simulink model "PPINFF"  (R2019a)
settings: Solver=VariableStepAuto  StartTime=0.0  StopTime=10.0  RelTol=1e-3
libraries: simulink x2
settings Model: Creator=pareshsoni  LastModifiedBy=pareshsoni

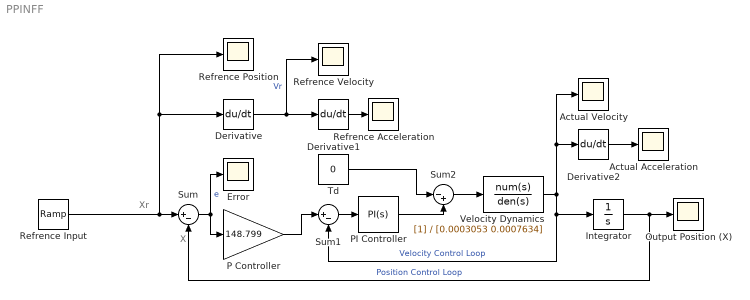
== system PPINFF ==
  note: X
  note: Xr
  Actual Acceleration : Scope
  Actual Velocity : Scope
  Derivative : Derivative  CoefficientInTFapproximation=0
  Derivative1 : Derivative
  Derivative2 : Derivative
  Error : Scope
  Integrator : Integrator
  Output Position (X) : Scope
  P Controller : Gain  Gain=148.799
  PI Controller : simulink/Continuous/PID Controller  Controller=PI  Form=Ideal  TimeDomain=Continuous-time  SampleTime=-1  IntegratorMethod=Forward Euler  FilterMethod=Forward Euler  ControllerParametersSource=internal  P=0.1296  I=25.1332  D=0  UseFilter=on  N=100  TunerSelectOption=Transfer Function Based (PID Tuner App)  InitialConditionSource=internal  InitialConditionForIntegrator=0  InitialConditionForFilter=0  DifferentiatorICPrevScaledInput=0  ExternalReset=none  TrackingMode=off  Kt=1  LimitOutput=off  UpperSaturationLimit=inf  LowerSaturationLimit=-inf  LinearizeAsGain=on  AntiWindupMode=none  Kb=1  POutMin=[]  POutMax=[]  IOutMin=[]  IOutMax=[]  DOutMin=[]  DOutMax=[]  NOutMin=[]  NOutMax=[]  SumOutMin=[]  SumOutMax=[]  SaturationOutMin=[]  SaturationOutMax=[]  PParamMin=[]  PParamMax=[]  IParamMin=[]  IParamMax=[]  DParamMin=[]  DParamMax=[]  NParamMin=[]  NParamMax=[]  KbParamMin=[]  KbParamMax=[]  KtParamMin=[]  KtParamMax=[]  KbOutMin=[]  KbOutMax=[]  KtOutMin=[]  KtOutMax=[]  IntegratorOutMin=[]  IntegratorOutMax=[]  FilterOutMin=[]  FilterOutMax=[]  SumI1OutMin=[]  SumI1OutMax=[]  SumI2OutMin=[]  SumI2OutMax=[]  SumI3OutMin=[]  SumI3OutMax=[]  SumI4OutMin=[]  SumI4OutMax=[]  SumDOutMin=[]  SumDOutMax=[]  DifferentiatorOutMin=[]  DifferentiatorOutMax=[]  FilterDiffOutCoefMin=[]  FilterDiffOutCoefMax=[]  ReciprocalOutMin=[]  ReciprocalOutMax=[]  SumDenOutMin=[]  SumDenOutMax=[]  SumNumOutMin=[]  SumNumOutMax=[]  DivideOutMin=[]  DivideOutMax=[]  IntegratorContinuousStateAttributes=''  IntegratorStateMustResolveToSignalObject=off  IntegratorRTWStateStorageClass=Auto  FilterContinuousStateAttributes=''  FilterStateMustResolveToSignalObject=off  FilterRTWStateStorageClass=Auto  ParallelPVariant=Passthrough  IdealPVariant=InternalParameters  IVariant=InternalParameters  DVariant=Disabled  IntegratorVariant=Continuous  SatVariant=Disabled  AWVariant=Passthrough  PCopyVariant=Disabled  TRVariant=Disabled  FdbkBlocksVariant=Forward  IdealPFdbkVariant=Disabled  SatFdbkVariant=Disabled  DerivativeFilterVariant=Disabled  NVariant=Disabled  NCopyVariant=Disabled_SignalSpec  FilterICVariant=Disabled  IntegratorICVariant=InternalICs  ExternalResetVariant=Disabled  TRSumVariant=Passthrough  SumFdbkVariant=Disabled  SumVariant=Sum_PI
  Refrence Acceleration : Scope
  Refrence Input : simulink/Sources/Ramp  slope=50  start=0  InitialOutput=0
  Refrence Position : Scope
  Refrence Velocity : Scope
  Sum : Sum  Inputs=|+-
  Sum1 : Sum  Inputs=|+-
  Sum2 : Sum  Inputs=|-+
  Td : Constant  Value=0
  Velocity Dynamics : TransferFcn  Denominator=[0.0003053 0.0007634]
  wires:
  Derivative/1 -> Refrence Velocity/1, Derivative1/1  "Vr"
  Derivative1/1 -> Refrence Acceleration/1
  Derivative2/1 -> Actual Acceleration/1
  Sum1/1 -> PI Controller/1
  Sum2/1 -> Velocity Dynamics/1
  PI Controller/1 -> Sum2/2
  Refrence Input/1 -> Sum/1, Refrence Position/1, Derivative/1
  P Controller/1 -> Sum1/1
  Sum/1 -> Error/1, P Controller/1  "e"
  Velocity Dynamics/1 -> Actual Velocity/1, Derivative2/1, Sum1/2, Integrator/1  "Velocity Control Loop"
  Integrator/1 -> Output Position (X)/1, Sum/2  "Position Control Loop"
  Td/1 -> Sum2/1
